simulink model "Rectangulo_sim"  (Simulink 7.1)
settings: Solver=ode45  StartTime=0.0  StopTime=10.0  RelTol=1e-3
undefined symbols (not defined in the file or in its folder): cinvMitsu, pol5Or_B, secuenciax
settings Model: Creator=Dario  LastModifiedBy=Dario

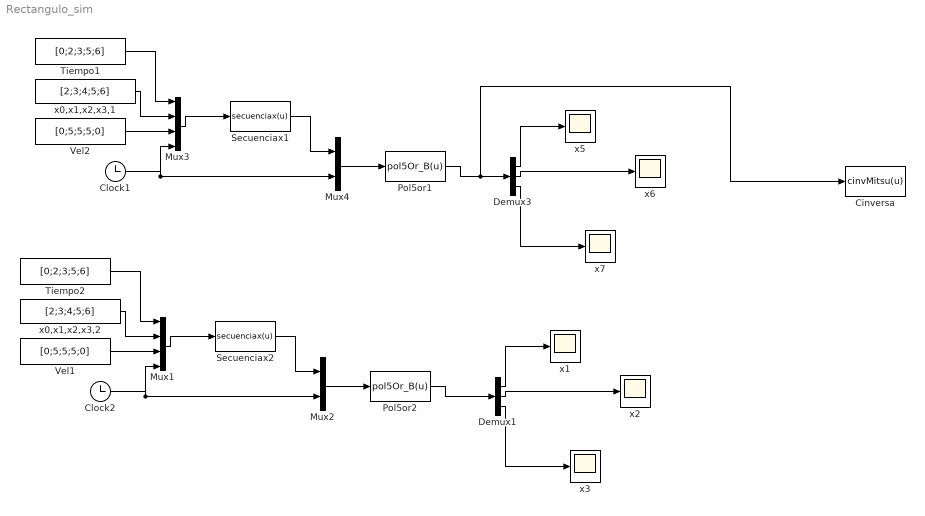
== system Rectangulo_sim ==
  Cinversa : MATLABFcn  MATLABFcn=cinvMitsu(u)  OutputDimensions=3
  Clock1 : Clock
      settings: Decimation=10
  Clock2 : Clock
      settings: Decimation=10
  Demux1 : Demux  Outputs=3
  Demux3 : Demux  Outputs=3
  Mux1 : Mux
  Mux2 : Mux  Inputs=2
  Mux3 : Mux
  Mux4 : Mux  Inputs=2
  Pol5or1 : MATLABFcn  MATLABFcn=pol5Or_B(u)  OutputDimensions=3
  Pol5or2 : MATLABFcn  MATLABFcn=pol5Or_B(u)  OutputDimensions=3
  Secuenciax1 : MATLABFcn  MATLABFcn=secuenciax(u)  OutputDimensions=6
  Secuenciax2 : MATLABFcn  MATLABFcn=secuenciax(u)  OutputDimensions=6
  Tiempo1 : Constant  Value=[0;2;3;5;6]  OutDataType=sfix(16)  OutScaling=2^0
  Tiempo2 : Constant  Value=[0;2;3;5;6]  OutDataType=sfix(16)  OutScaling=2^0
  Vel1 : Constant  Value=[0;5;5;5;0]  OutDataType=sfix(16)  OutScaling=2^0
  Vel2 : Constant  Value=[0;5;5;5;0]  OutDataType=sfix(16)  OutScaling=2^0
  x0,x1,x2,x3,1 : Constant  Value=[2;3;4;5;6]  OutDataType=sfix(16)  OutScaling=2^0
  x0,x1,x2,x3,2 : Constant  Value=[2;3;4;5;6]  OutDataType=sfix(16)  OutScaling=2^0
  x{1..3,5..7} (6 alike) : Scope
      x2 settings: SaveName=ScopeData4
      x3 settings: SaveName=ScopeData5
      x6 settings: SaveName=ScopeData2
      x7 settings: SaveName=ScopeData3
  wires:
  Mux3/1 -> Secuenciax1/1
  Tiempo1/1 -> Mux3/1
  x0,x1,x2,x3,1/1 -> Mux3/2
  Clock1/1 -> Mux3/4, Mux4/2
  Mux4/1 -> Pol5or1/1
  Vel2/1 -> Mux3/3
  Secuenciax1/1 -> Mux4/1
  Pol5or1/1 -> Demux3/1, Cinversa/1
  Demux3/1 -> x5/1
  Demux3/2 -> x6/1
  Demux3/3 -> x7/1
  Mux1/1 -> Secuenciax2/1
  Tiempo2/1 -> Mux1/1
  x0,x1,x2,x3,2/1 -> Mux1/2
  Clock2/1 -> Mux1/4, Mux2/2
  Mux2/1 -> Pol5or2/1
  Vel1/1 -> Mux1/3
  Secuenciax2/1 -> Mux2/1
  Pol5or2/1 -> Demux1/1
  Demux1/1 -> x1/1
  Demux1/2 -> x2/1
  Demux1/3 -> x3/1
